simulink model "FOC_MIL_"  (R2020b)
settings: Solver=FixedStepAuto  StartTime=0.0  StopTime=6  FixedStep=Ts  RelTol=1e-3
values from neighbouring files (symbols this model uses):
  Tctr = 0.0000625    (= 6.25e-05)    [FOC_Config.m]
  Ts = 0.0001    [FOC_Config.m]
undefined symbols (not defined in the file or in its folder): motor
libraries: mcbplantlib x1, autolibpmsminterior x1
settings Model: Creator=k  LastModifiedBy=k

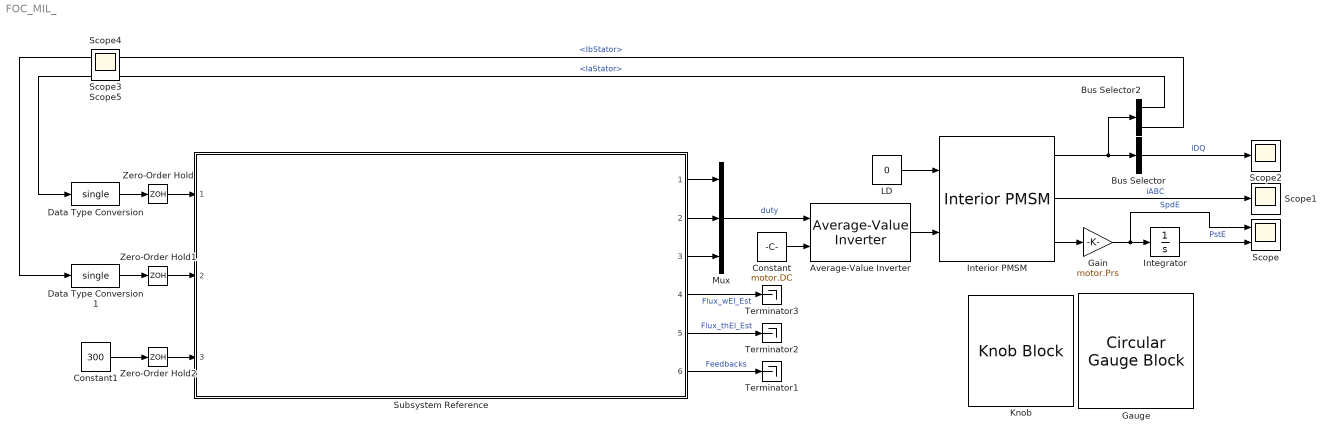
== system FOC_MIL_ ==
  Average-Value Inverter : mcbplantlib/Average-Value Inverter
  Bus Selector : BusSelector  OutputSignals=IdSync,IqSync  OutputAsBus=on
  Bus Selector2 : BusSelector  OutputSignals=IaStator,IbStator
  Constant : Constant  Value=motor.DC
  Constant1 : Constant  Value=300  OutDataTypeStr=single
  Data Type Conversion : DataTypeConversion  OutDataTypeStr=single
  Data Type Conversion1 : DataTypeConversion  OutDataTypeStr=single
  Gain : Gain  Gain=motor.Prs
  Gauge : CircularGaugeBlock  ScaleMax=6.28  TickInterval=1.57
  Integrator : Integrator  WrapState=on  WrappedStateUpperValue=2*pi  WrappedStateLowerValue=0
  Interior PMSM : autolibpmsminterior/Interior PMSM  port_config=Torque  sim_type=Continuous  Ts=Ts  P=motor.Prs  Rs=motor.Rs  Ldq=[motor.Ld motor.Lq]  KConstText=Permanent flux linkage constant (lambda_pm):  lambda_pm=motor.Flux  Ke=159.9771  mechanical=[motor.J, motor.B, motor.Tf]  idq0=[0 0]  theta_init=0  omega_init=0  KConst=motor.Flux  lambda_pm_calc=motor.Flux  Kt=0.07  RefBlkName='autolibpmsminterior/Interior PMSM'  aMode=5
      settings: SourceProductBaseCode=PW,MT,UV,VE,VP
  Knob : KnobBlock  ScaleMin=100  ScaleMax=400
  LD : Constant  Value=0
  Mux : Mux  Inputs=3
  Scope : Scope  NumInputPorts=2
  Scope{1..5} (5 alike) : Scope
  Subsystem Reference : Subsystem  ReferencedSubsystem=FOC_Algoithm_Model
  Terminator1 : Terminator
  Terminator2 : Terminator
  Terminator3 : Terminator
  Zero-Order Hold : ZeroOrderHold  SampleTime=Tctr
  Zero-Order Hold1 : ZeroOrderHold  SampleTime=Tctr
  Zero-Order Hold2 : ZeroOrderHold  SampleTime=Tctr
  wires:
  Integrator/1 -> Scope/2  "PstE"
  Subsystem Reference/3 -> Mux/3
  Bus Selector/1 -> Scope2/1  "iDQ"
  LD/1 -> Interior PMSM/1
  Interior PMSM/1 -> Bus Selector/1, Bus Selector2/1
  Subsystem Reference/2 -> Mux/2
  Gain/1 -> Integrator/1, Scope/1  "SpdE"
  Interior PMSM/2 -> Scope1/1  "iABC"
  Subsystem Reference/1 -> Mux/1
  Interior PMSM/3 -> Gain/1
  Bus Selector2/1 -> Data Type Conversion/1  "<IaStator>"
  Bus Selector2/2 -> Data Type Conversion1/1  "<IbStator>"
  Data Type Conversion/1 -> Zero-Order Hold/1
  Data Type Conversion1/1 -> Zero-Order Hold1/1
  Zero-Order Hold/1 -> Subsystem Reference/1
  Zero-Order Hold1/1 -> Subsystem Reference/2
  Constant/1 -> Average-Value Inverter/2
  Mux/1 -> Average-Value Inverter/1  "duty"
  Average-Value Inverter/1 -> Interior PMSM/2
  Subsystem Reference/5 -> Terminator2/1  "Flux_thEl_Est"
  Subsystem Reference/4 -> Terminator3/1  "Flux_wEl_Est"
  Constant1/1 -> Zero-Order Hold2/1
  Subsystem Reference/6 -> Terminator1/1  "Feedbacks"
  Zero-Order Hold2/1 -> Subsystem Reference/3
